simulink model "CLLC_converter_switching_model_closed_loop"  (R2021a)
settings: Solver=VariableStepAuto  StartTime=0.0  StopTime=10.0  MaxStep=1e-9  RelTol=1e-3
undefined symbols (not defined in the file or in its folder): Ion, Lithium
libraries: spsSeriesRLCBranchLib x26, spsMosfetLib x8, spsVoltageMeasurementLib x7, spsCurrentMeasurementLib x6, spsControlledVoltageSourceLib x5, pid_lib x2, spsBatteryLib x1, spsLinearTransformerLib x1, simulink x1, spsVariableResistorLib x1, spspowerguiLib x1
settings Model: Creator=prizm  LastModifiedBy=prizm
settings RTWCC: GenCodeOnly=on

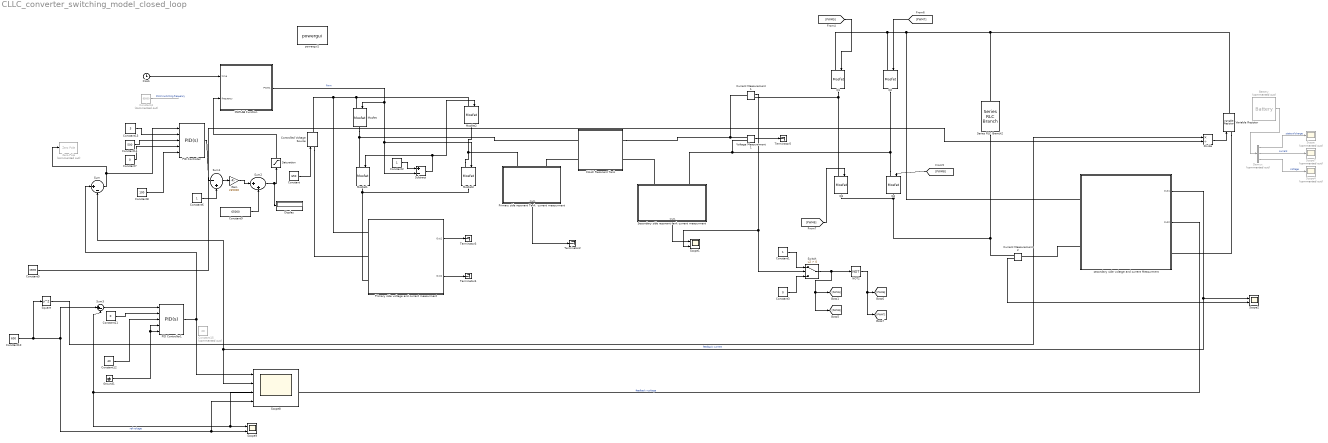
== system CLLC_converter_switching_model_closed_loop ==
  Battery : spsBatteryLib/Battery  Commented=on  BatType=Lithium-Ion  ShowTempParam=off  ThermalPreset=no  ShowAgeParam=off  NomV=662  NomQ=500  SOC=60  Batt_Tr=5e-3  PresetModel=on  MaxQ=500  MinV=496.5  FullV=770.5595  Dis_rate=217.3913  R=0.01324  Normal_OP=452.1739  expZone="[715.2154      24.56522]"  current=[6.5 13 32.5]  Units=Time  Tci=20  NomT=20  T2=-30  MaxQ2=4.8  FullV2=7.1  Normal_OP2=5.655  expZone2="[6.58           1]"  Rca=0.6  ti=2000  Dp=0  Neq0=0  Tsim=1e6  Ta1=25  Qeol=5.4*0.9  Reol=0.013333*1.2  Char_age=[2.3478, 3]  Dis_age=[2.3478, 10]  N1=1500  N2=10500  N3=1000  N4=1400  Ta2=45  N5=950
  "CLLLC Resonant Tank " : Subsystem
  Clock : Clock
  Constant : Constant  Value=650
  Constant1 : Constant
  Constant10 : Constant  Value=600
  Constant11 : Constant  Value=0
  Constant12 : Constant  Value=40
  Constant13 : Constant  Value=3
  Constant14 : Constant  Value=500
  Constant15 : Constant  Commented=on  Value=20  SampleTime=1e-9
  Constant2 : Constant
  Constant3 : Constant  Value=0
  Constant4 : Constant  Commented=on  Value=65000
  Constant5 : Constant  Value=15000  SampleTime=1e-9
  Constant6 : Constant
  Constant7 : Constant  Value=0
  Constant8 : Constant  Value=100
  Constant9 : Constant  Value=65000
  Controlled Voltage Source : spsControlledVoltageSourceLib/Controlled Voltage Source  Initialize=on  Source_Type=DC  Amplitude=0  Phase=0  Frequency=0  Measurements=None
  Current Measurement1 : spsCurrentMeasurementLib/Current Measurement  PhasorSimulation=off  OutputType=Complex  PSBequivalent=0
  Current Measurement2 : spsCurrentMeasurementLib/Current Measurement  PhasorSimulation=off  OutputType=Complex  PSBequivalent=0
  Demux : Demux  Commented=on  Outputs=3
  Display : Display
  Divide : Product  Inputs=*/
  Gain : Gain  Gain=235000
  Ground1 : Ground
  MATLAB Function : MATLAB Function  TreatAsAtomicUnit=on
  Mosfet{,1..3} (4 alike) : spsMosfetLib/Mosfet  Ron=0.1  Lon=0  Rd=0.01  Vfd=2  IC=0  Rs=1e5  Cs=inf  Measurements=off
  NOT2 : Logic  Operator=NOT  IconShape=distinctive  AllPortsSameDT=off  OutDataTypeStr=boolean
  PID Controller : pid_lib/PID Controller  Controller=PID  Form=Parallel  TimeDomain=Continuous-time  UseExternalTs=off  SampleTime=-1  IntegratorMethod=Forward Euler  FilterMethod=Forward Euler  ControllerParametersSource=external  P=0.00014927  I=100  D=0  UseFilter=on  N=100  TunerSelectOption=Frequency Response Based  InitialConditionSource=internal  InitialConditionForIntegrator=0  InitialConditionForFilter=0  DifferentiatorICPrevScaledInput=0  ExternalReset=none  TrackingMode=off  Kt=1  LimitOutput=on  SatLimitsSource=internal  UpperSaturationLimit=1  LowerSaturationLimit=0  LinearizeAsGain=on  AntiWindupMode=clamping  Kb=1  POutMin=[]  POutMax=[]  IOutMin=[]  IOutMax=[]  DOutMin=[]  DOutMax=[]  NOutMin=[]  NOutMax=[]  SumOutMin=[]  SumOutMax=[]  SaturationOutMin=[]  SaturationOutMax=[]  PParamMin=[]  PParamMax=[]  IParamMin=[]  IParamMax=[]  DParamMin=[]  DParamMax=[]  NParamMin=[]  NParamMax=[]  KbParamMin=[]  KbParamMax=[]  KtParamMin=[]  KtParamMax=[]  KbOutMin=[]  KbOutMax=[]  KtOutMin=[]  KtOutMax=[]  IntegratorOutMin=[]  IntegratorOutMax=[]  FilterOutMin=[]  FilterOutMax=[]  SumI1OutMin=[]  SumI1OutMax=[]  SumI2OutMin=[]  SumI2OutMax=[]  SumI3OutMin=[]  SumI3OutMax=[]  SumI4OutMin=[]  SumI4OutMax=[]  SumDOutMin=[]  SumDOutMax=[]  DifferentiatorOutMin=[]  DifferentiatorOutMax=[]  FilterDiffOutCoefMin=[]  FilterDiffOutCoefMax=[]  ReciprocalOutMin=[]  ReciprocalOutMax=[]  SumDenOutMin=[]  SumDenOutMax=[]  SumNumOutMin=[]  SumNumOutMax=[]  DivideOutMin=[]  DivideOutMax=[]  UdiffTsProdOutMin=[]  UdiffTsProdOutMax=[]  NTsProdOutMin=[]  NTsProdOutMax=[]  UintegralTsProdOutMin=[]  UintegralTsProdOutMax=[]  UngainTsProdOutMin=[]  UngainTsProdOutMax=[]  IntegratorContinuousStateAttributes=''  IntegratorStateMustResolveToSignalObject=off  IntegratorRTWStateStorageClass=Auto  FilterContinuousStateAttributes=''  FilterStateMustResolveToSignalObject=off  FilterRTWStateStorageClass=Auto  ParallelPVariant=ExternalParameters  IdealPVariant=Disabled  IVariant=ExternalParameters  DVariant=ExternalParameters  IntegratorVariant=Continuous  SatVariant=Enabled  AWVariant=ContClampingParallel  PCopyVariant=Disabled  TRVariant=Disabled  FdbkBlocksVariant=Forward  IdealPFdbkVariant=Disabled  SatFdbkVariant=Disabled  DerivativeFilterVariant=ContFilter  NVariant=ExternalParameters  NCopyVariant=Disabled  FilterICVariant=InternalICsFilter  IntegratorICVariant=InternalICs  ExternalResetVariant=Disabled  TRSumVariant=Passthrough  SumFdbkVariant=Disabled  SumVariant=Sum_PID  TsampFilterVariant=InternalTs  TsampNgainVariant=Passthrough  TsampIntegralVariant=Passthrough  ExternalSaturationOutDataTypeStr=Inherit: Same as second input
  PID Controller1 : pid_lib/PID Controller  Controller=PID  Form=Parallel  TimeDomain=Continuous-time  UseExternalTs=off  SampleTime=-1  IntegratorMethod=Forward Euler  FilterMethod=Forward Euler  ControllerParametersSource=external  P=0.00014927  I=100  D=0  UseFilter=on  N=100  TunerSelectOption=Frequency Response Based  InitialConditionSource=internal  InitialConditionForIntegrator=0  InitialConditionForFilter=0  DifferentiatorICPrevScaledInput=0  ExternalReset=none  TrackingMode=off  Kt=1  LimitOutput=on  SatLimitsSource=internal  UpperSaturationLimit=30  LowerSaturationLimit=5  LinearizeAsGain=on  AntiWindupMode=clamping  Kb=1  POutMin=[]  POutMax=[]  IOutMin=[]  IOutMax=[]  DOutMin=[]  DOutMax=[]  NOutMin=[]  NOutMax=[]  SumOutMin=[]  SumOutMax=[]  SaturationOutMin=[]  SaturationOutMax=[]  PParamMin=[]  PParamMax=[]  IParamMin=[]  IParamMax=[]  DParamMin=[]  DParamMax=[]  NParamMin=[]  NParamMax=[]  KbParamMin=[]  KbParamMax=[]  KtParamMin=[]  KtParamMax=[]  KbOutMin=[]  KbOutMax=[]  KtOutMin=[]  KtOutMax=[]  IntegratorOutMin=[]  IntegratorOutMax=[]  FilterOutMin=[]  FilterOutMax=[]  SumI1OutMin=[]  SumI1OutMax=[]  SumI2OutMin=[]  SumI2OutMax=[]  SumI3OutMin=[]  SumI3OutMax=[]  SumI4OutMin=[]  SumI4OutMax=[]  SumDOutMin=[]  SumDOutMax=[]  DifferentiatorOutMin=[]  DifferentiatorOutMax=[]  FilterDiffOutCoefMin=[]  FilterDiffOutCoefMax=[]  ReciprocalOutMin=[]  ReciprocalOutMax=[]  SumDenOutMin=[]  SumDenOutMax=[]  SumNumOutMin=[]  SumNumOutMax=[]  DivideOutMin=[]  DivideOutMax=[]  UdiffTsProdOutMin=[]  UdiffTsProdOutMax=[]  NTsProdOutMin=[]  NTsProdOutMax=[]  UintegralTsProdOutMin=[]  UintegralTsProdOutMax=[]  UngainTsProdOutMin=[]  UngainTsProdOutMax=[]  IntegratorContinuousStateAttributes=''  IntegratorStateMustResolveToSignalObject=off  IntegratorRTWStateStorageClass=Auto  FilterContinuousStateAttributes=''  FilterStateMustResolveToSignalObject=off  FilterRTWStateStorageClass=Auto  ParallelPVariant=ExternalParameters  IdealPVariant=Disabled  IVariant=ExternalParameters  DVariant=ExternalParameters  IntegratorVariant=Continuous  SatVariant=Enabled  AWVariant=ContClampingParallel  PCopyVariant=Disabled  TRVariant=Disabled  FdbkBlocksVariant=Forward  IdealPFdbkVariant=Disabled  SatFdbkVariant=Disabled  DerivativeFilterVariant=ContFilter  NVariant=ExternalParameters  NCopyVariant=Disabled  FilterICVariant=InternalICsFilter  IntegratorICVariant=InternalICs  ExternalResetVariant=Disabled  TRSumVariant=Passthrough  SumFdbkVariant=Disabled  SumVariant=Sum_PID  TsampFilterVariant=InternalTs  TsampNgainVariant=Passthrough  TsampIntegralVariant=Passthrough  ExternalSaturationOutDataTypeStr=Inherit: Same as second input
  "Primary side resonant Tank  current measurment " : Subsystem
  "Primary side voltage and current measurment " : Subsystem
  Q{1..4} (4 alike) : spsMosfetLib/Mosfet  Ron=0.1  Lon=0  Rd=0.01  Vfd=2  IC=0  Rs=1e5  Cs=inf  Measurements=off
  Saturation : Saturate  UpperLimit=300000  LowerLimit=60000
  Scope : Scope  Commented=on
  Scope1 : Scope  NumInputPorts=2
  Scope2 : Scope  NumInputPorts=2
  Scope4 : Scope  Commented=on
  Scope7 : Scope  Commented=on
  Scope8 : Scope  NumInputPorts=4
  Scope9 : Scope  NumInputPorts=2
  "Secondary side resonant tank current measurment " : Subsystem
  Series RLC Branch2 : spsSeriesRLCBranchLib/Series RLC Branch  LConnTagsString=__new0  RConnTagsString=__new0  BranchType=C  Resistance=54.0  Inductance=0.2533e-3  SetiL0=off  InitialCurrent=0  Capacitance=10e-6  Setx0=off  InitialVoltage=0  Measurements=None
  Square : Math  Operator=square  SaturateOnIntegerOverflow=on
  Subtract : Sum  Inputs=+-
  Sum : Sum  Inputs=|+-
  Sum1 : Sum  Inputs=|-+
  Sum2 : Sum  Inputs=|++
  Sum3 : Sum  Inputs=|+-
  Switch : Switch  Criteria=u2 > Threshold
  Terminator{2..5} (4 alike) : Terminator
  Variable Resistor : spsVariableResistorLib/Variable Resistor  Rabsmin=1e-3
      settings: SourceProductBaseCode=PS
  Voltage Measurement1 : spsVoltageMeasurementLib/Voltage Measurement  PhasorSimulation=off  OutputType=Complex  PSBequivalent=0
  Zero-Pole : ZeroPole  Commented=on  Zeros=[-3.48e4 -3.48e4]  Poles=[0 -5e4 -3.7699e5]  Gain=[600]
  powergui1 : spspowerguiLib/powergui  Priority=1  SimulationMode=Discrete  SampleTime=1e-9  frequency=60  Iterations=50  frequencyindice=0  Pbase=100e6  ErrMax=1e-4  UnitsV=kV  UnitsW=MW  buscounter=0  FunctionMessages=off  echomessages=off  EnableUseOfTLC=off  CurrentSourceSwitches=off  DisableSnubberDevices=off  DisableRonSwitches=off  DisableVfSwitches=off  DisplayEquations=off  AutomaticDiscreteSolvers=off  SolverType=Tustin/Backward Euler (TBE)  Interpol=off  ExternalGateDelay=off  methode=off  Ts=100  x0status=blocks  SPID=on  SwTol=0  HookPort=off  NonlinearTolerance=1e-4  nMaxIteration=100  ContinueOnMaxIteration=off  RestoreLinks=warning  ResistiveCurrentMeasurement=off  Frange=[0:2:500]  Ylog=off  Xlog=on  ShowGrid=off  save=off  variable=ZData  structure=0  ZoomFFT=off  StartTime=0.0  cycles=1  DisplayStyle=1  fundamental=60  FreqAxis=off  MaxFrequency=1000  frequencyindicesteady=1  RmsSteady=1  display=off
  "secondary side volatge and current Measurment " : Subsystem
  wires:
  Constant/1 -> Controlled Voltage Source/1
  MATLAB Function/1(PWM1) -> Mosfet/1, Mosfet3/1, Subtract/2  "Pwm"
  Constant2/1 -> Subtract/1
  Subtract/1 -> Mosfet2/1, Mosfet1/1
  [PWM7] -> Q2/1
  [PWM6] -> Q3/1
  [PWM8] -> Q4/1
  [PWM5] -> Q1/1
  NOT2/1 -> [PWM6], [PWM7]
  Switch/1 -> [PWM5], [PWM8], NOT2/1
  Current Measurement1/1 -> Scope1/2, Switch/2
  Constant3/1 -> Switch/3
  Constant1/1 -> Switch/1
  Voltage Measurement1/1 -> Terminator5/1
  Sum/1 -> PID Controller/1, Zero-Pole/1
  Constant9/1 -> Sum2/2
  Sum2/1 -> Display/1, Saturation/1
  Ground1/1 -> PID Controller1/5, PID Controller1/4
  Constant10/1 -> Square/1, Sum3/1, Scope8/4, Scope9/2  "ref voltage"
  Sum3/1 -> PID Controller1/1
  Constant11/1 -> PID Controller1/2
  Constant12/1 -> PID Controller1/3
  Sum1/1 -> Gain/1
  Constant6/1 -> Sum1/2
  Saturation/1 -> MATLAB Function/2(frequency)
  Gain/1 -> Sum2/1
  Constant13/1 -> PID Controller/2
  Constant14/1 -> PID Controller/3
  Constant4/1 -> ?  "PWM switching frequency"
  Clock/1 -> MATLAB Function/1(time)
  "Primary side voltage and current measurment "/1(Out1) -> Terminator3/1
  "Primary side voltage and current measurment "/2(Out2) -> Terminator4/1
  "Primary side resonant Tank  current measurment "/1(Out1) -> Terminator2/1
  "Secondary side resonant tank current measurment "/1(Out1) -> Scope1/1
  "secondary side volatge and current Measurment "/2(Out2) -> Sum3/2, Scope8/3, Scope9/1  "feedback vcoltage"
  "secondary side volatge and current Measurment "/1(Out1) -> Scope2/1, Sum/2, Scope8/2  "feedback current"
  Battery/1 -> Demux/1
  Demux/1 -> Scope/1  "state of charge"
  Demux/2 -> Scope7/1  "current"
  Demux/3 -> Scope4/1  "Voltage"
  PID Controller/1 -> Sum1/1
  Constant7/1 -> PID Controller/4
  Constant8/1 -> PID Controller/5
  Divide/1 -> Variable Resistor/1
  PID Controller1/1 -> Sum/1, Scope8/1
  Constant5/1 -> Divide/2
  Square/1 -> Divide/1
  Current Measurement2/1 -> Scope2/2
  connections:
  Controlled Voltage Source/RConn1 -- "Primary side voltage and current measurment "/LConn1 -- Mosfet/LConn1 -- Mosfet2/LConn1
  Mosfet3/RConn1 -- "Primary side voltage and current measurment "/LConn3 -- Mosfet1/RConn1
  Q1/RConn1 -- Q3/LConn1 -- Current Measurement1/RConn1
  Voltage Measurement1/LConn1 -- Current Measurement1/LConn1 -- "CLLLC Resonant Tank "/RConn1
  Controlled Voltage Source/LConn1 -- "Primary side voltage and current measurment "/LConn2
  Mosfet3/LConn1 -- Mosfet2/RConn1 -- "Primary side resonant Tank  current measurment "/LConn1
  Q4/LConn1 -- Q2/RConn1 -- Voltage Measurement1/LConn2 -- "Secondary side resonant tank current measurment "/LConn2
  Q2/LConn1 -- Q1/LConn1 -- Variable Resistor/RConn1 -- Series RLC Branch2/LConn1 -- "secondary side volatge and current Measurment "/LConn1
  Q3/RConn1 -- Current Measurement2/RConn1 -- Series RLC Branch2/RConn1 -- Q4/RConn1
  Variable Resistor/LConn1 -- "secondary side volatge and current Measurment "/RConn1
  Mosfet/RConn1 -- Mosfet1/LConn1 -- "CLLLC Resonant Tank "/LConn1
  "Primary side resonant Tank  current measurment "/LConn2 -- "CLLLC Resonant Tank "/LConn2
  "Secondary side resonant tank current measurment "/LConn1 -- "CLLLC Resonant Tank "/RConn2
  "secondary side volatge and current Measurment "/LConn2 -- Current Measurement2/LConn1

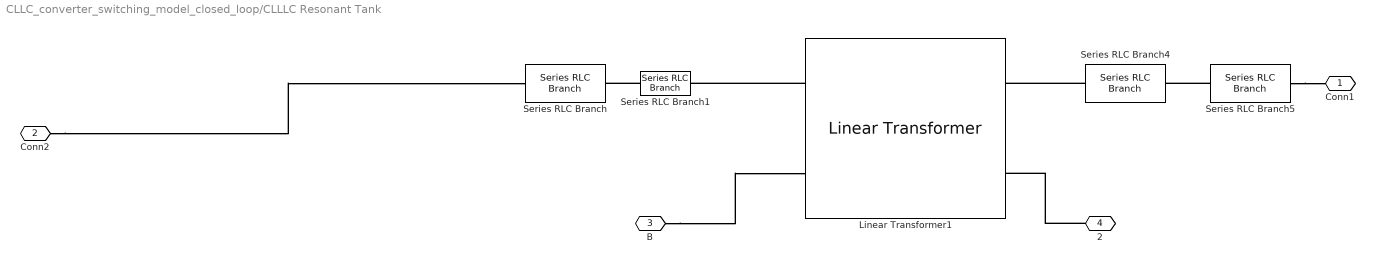
== system CLLC_converter_switching_model_closed_loop/CLLLC Resonant Tank  ==
  Linear Transformer1 : spsLinearTransformerLib/Linear Transformer  UNITS=SI  NominalPower=[15000 60000]  winding1=[500 0.003 10e-9]  winding2=[650 0.003 10e-9]  ThreeWindings=off  winding3=[3.15e+05 0 0]  RmLm=[10e9 100e-6]  Measurements=None  DataType=on
  Series RLC Branch : spsSeriesRLCBranchLib/Series RLC Branch  LConnTagsString=__new0  RConnTagsString=__new0  BranchType=C  Resistance=1  Inductance=1e-3  SetiL0=off  InitialCurrent=0  Capacitance=300e-9  Setx0=off  InitialVoltage=0  Measurements=None
  Series RLC Branch1 : spsSeriesRLCBranchLib/Series RLC Branch  LConnTagsString=__new0  RConnTagsString=__new0  BranchType=L  Resistance=1  Inductance=20e-6  SetiL0=off  InitialCurrent=0  Capacitance=1e-6  Setx0=off  InitialVoltage=0  Measurements=None
  Series RLC Branch4 : spsSeriesRLCBranchLib/Series RLC Branch  LConnTagsString=__new0  RConnTagsString=__new0  BranchType=L  Resistance=1  Inductance=20e-6  SetiL0=off  InitialCurrent=0  Capacitance=1e-6  Setx0=off  InitialVoltage=0  Measurements=None
  Series RLC Branch5 : spsSeriesRLCBranchLib/Series RLC Branch  LConnTagsString=__new0  RConnTagsString=__new0  BranchType=C  Resistance=1  Inductance=1e-3  SetiL0=off  InitialCurrent=0  Capacitance=480e-9  Setx0=off  InitialVoltage=0  Measurements=None
  Conn1 : PMIOPort  Side=Right
  Conn2 : PMIOPort  Port=2  Side=Left
  B : PMIOPort  Port=3  Side=Left
  2 : PMIOPort  Port=4  Side=Right
  connections:
  Linear Transformer1/LConn1 -- Series RLC Branch1/RConn1
  Series RLC Branch5/LConn1 -- Series RLC Branch4/LConn1
  Series RLC Branch1/LConn1 -- Series RLC Branch/RConn1
  Conn2/RConn1 -- Series RLC Branch/LConn1
  B/RConn1 -- Linear Transformer1/LConn2
  2/RConn1 -- Linear Transformer1/RConn2
  Series RLC Branch4/RConn1 -- Linear Transformer1/RConn1
  Series RLC Branch5/RConn1 -- Conn1/RConn1

== system CLLC_converter_switching_model_closed_loop/Primary side resonant Tank  current measurment  ==
  ADC conversion to bits  2 : Subsystem
  CLLLC primary side  side current measurment 2 : Subsystem
  conversion from bits to current1 : Subsystem
  - : PMIOPort  Side=Left
  + : PMIOPort  Port=2  Side=Left
  Out1 : Outport
  wires:
  ADC conversion to bits  2/1(reference) -> conversion from bits to current1/1(reference)
  CLLLC primary side  side current measurment 2/1(v) -> ADC conversion to bits  2/1(v)
  ADC conversion to bits  2/2(Out2) -> conversion from bits to current1/2(In2)
  conversion from bits to current1/1(Out1) -> Out1/1
  connections:
  -/RConn1 -- CLLLC primary side  side current measurment 2/LConn1
  CLLLC primary side  side current measurment 2/LConn2 -- +/RConn1

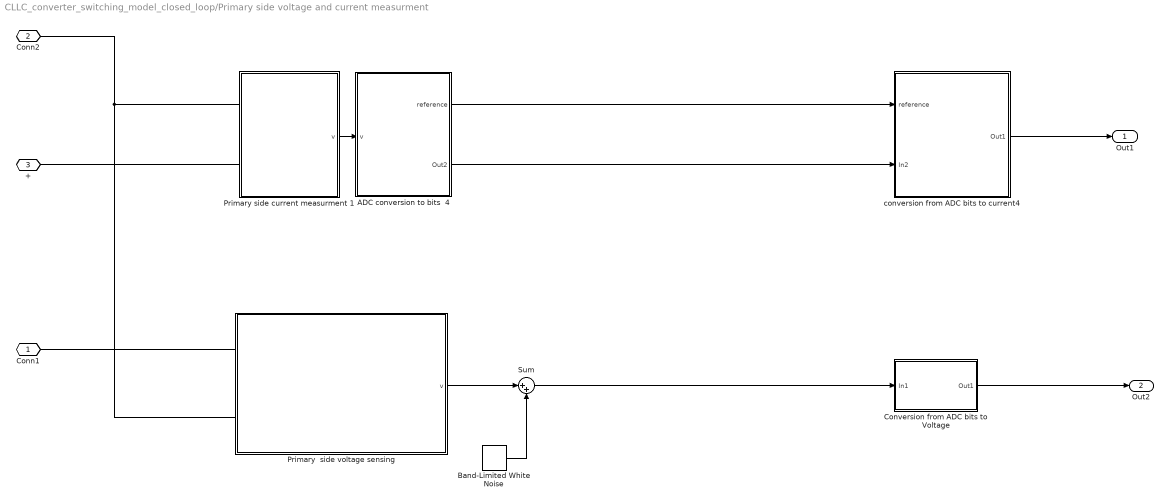
== system CLLC_converter_switching_model_closed_loop/Primary side voltage and current measurment  ==
  ADC conversion to bits  4 : Subsystem
  Band-Limited White Noise : simulink/Sources/Band-Limited White Noise  Cov=[0.1]  Ts=1e-4  seed=[23341]
  "Conversion from ADC bits to Voltage " : Subsystem
  "Primary  side voltage sensing " : Subsystem
  Primary side current measurment 1 : Subsystem
  Sum : Sum  Inputs=|++
  conversion from ADC bits to current4 : Subsystem
  Conn1 : PMIOPort  Side=Left
  Conn2 : PMIOPort  Port=2  Side=Left
  + : PMIOPort  Port=3  Side=Left
  Out1 : Outport
  Out2 : Outport  Port=2
  wires:
  ADC conversion to bits  4/2(Out2) -> conversion from ADC bits to current4/2(In2)
  Primary side current measurment 1/1(v) -> ADC conversion to bits  4/1(v)
  conversion from ADC bits to current4/1(Out1) -> Out1/1
  ADC conversion to bits  4/1(reference) -> conversion from ADC bits to current4/1(reference)
  "Primary  side voltage sensing "/1(v) -> Sum/1
  Band-Limited White Noise/1 -> Sum/2
  Sum/1 -> "Conversion from ADC bits to Voltage "/1(In1)
  "Conversion from ADC bits to Voltage "/1(Out1) -> Out2/1
  connections:
  Conn1/RConn1 -- "Primary  side voltage sensing "/LConn1
  Primary side current measurment 1/LConn2 -- +/RConn1
  Primary side current measurment 1/LConn1 -- Conn2/RConn1 -- "Primary  side voltage sensing "/LConn2

== system CLLC_converter_switching_model_closed_loop/Secondary side resonant tank current measurment  ==
  ADC conversion to bits  1 : Subsystem
  "CLLLC secondary side current measurment " : Subsystem
  conversion from bits to current2 : Subsystem
  - : PMIOPort  Side=Left
  + : PMIOPort  Port=2  Side=Left
  Out1 : Outport
  wires:
  "CLLLC secondary side current measurment "/1(v) -> ADC conversion to bits  1/1(v)
  ADC conversion to bits  1/2(Out2) -> conversion from bits to current2/2(In2)
  ADC conversion to bits  1/1(reference) -> conversion from bits to current2/1(reference)
  conversion from bits to current2/1(Out1) -> Out1/1
  connections:
  "CLLLC secondary side current measurment "/LConn1 -- -/RConn1
  +/RConn1 -- "CLLLC secondary side current measurment "/LConn2

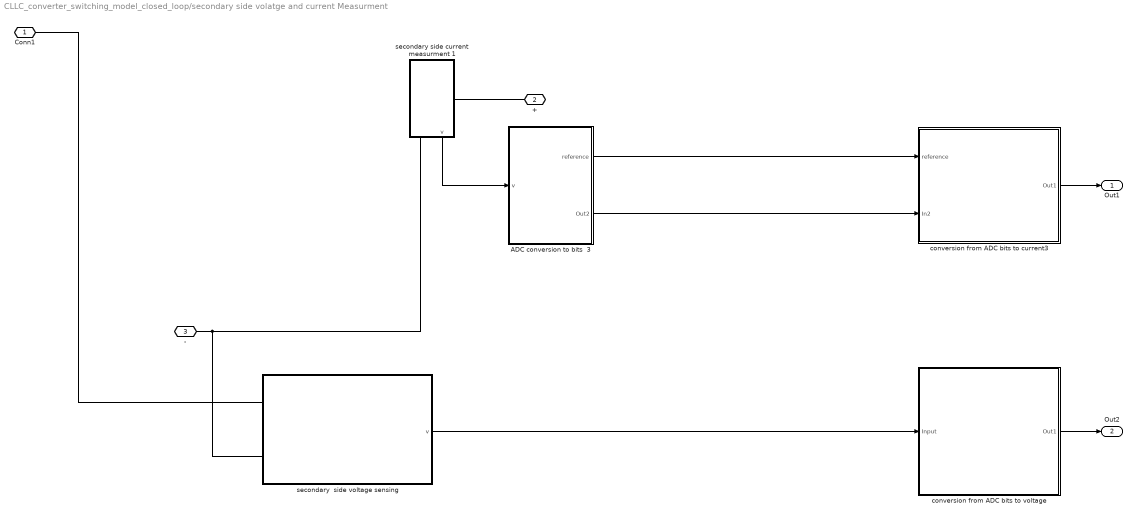
== system CLLC_converter_switching_model_closed_loop/secondary side volatge and current Measurment  ==
  ADC conversion to bits  3 : Subsystem
  conversion from ADC bits to current3 : Subsystem
  "conversion from ADC bits to voltage " : Subsystem
  "secondary  side voltage sensing " : Subsystem
  secondary side current measurment 1 : Subsystem
      settings: PortSchema="{\"entries\":[{\"content\":{\"sides\":[{\"content\":{\"connectorIds\":[]},\"type\":\"ConnectorPlacement.EquallySpacedRectSide\",\"uuid\":\"6682aabd-b4c9-4e26-ac42-b7f4937c9882\"},{\"content\":{\"connectorIds\":[\"RConn1\",\"Out1\"],\"side\":\"RIGHT\"},\"type\":\"ConnectorPlacement.EquallySpacedRectSide\",\"uuid\":\"39693c9e-f70a-4c1a-90ac-326607627fb7\"},{\"content\":{\"connectorIds\":[],\"side\":\"TOP\"},\"type\":\"ConnectorPlacement.EquallySpacedRectSide\",\"uuid\":\"8ffbc9bf-ac02-4293-be03-d78ae118879d\"},{\"content\":{\"connectorIds\":[\"RConn2\"],\"side\":\"BOTTOM\"},\"type\":\"ConnectorPlacement.EquallySpacedRectSide\",\"uuid\":\"c1ea8c00-373b-4bbb-8642-07b7e9a91a0c\"}]},\"type\":\"ConnectorPlacement.EquallySpacedConnector\",\"uuid\":\"fc66d08e-e92c-4509-bb77-625124f73eef\"}],\"packageUris\":[\"http://schema.mathworks.com/mf0/Connector/R2020b\"],\"version\":\"1.0\"}"
  Conn1 : PMIOPort  Side=Left
  + : PMIOPort  Port=2  Side=Right
  - : PMIOPort  Port=3  Side=Left
  Out1 : Outport
  Out2 : Outport  Port=2
  wires:
  secondary side current measurment 1/1(v) -> ADC conversion to bits  3/1(v)
  ADC conversion to bits  3/2(Out2) -> conversion from ADC bits to current3/2(In2)
  ADC conversion to bits  3/1(reference) -> conversion from ADC bits to current3/1(reference)
  conversion from ADC bits to current3/1(Out1) -> Out1/1
  "secondary  side voltage sensing "/1(v) -> "conversion from ADC bits to voltage "/1(Input)
  "conversion from ADC bits to voltage "/1(Out1) -> Out2/1
  connections:
  Conn1/RConn1 -- "secondary  side voltage sensing "/LConn1
  +/RConn1 -- secondary side current measurment 1/RConn2
  -/RConn1 -- "secondary  side voltage sensing "/LConn2 -- secondary side current measurment 1/RConn1

== system CLLC_converter_switching_model_closed_loop/Primary side resonant Tank  current measurment /ADC conversion to bits  2 ==
  v : Inport
  Gain3 : Gain  Gain=(2^12)/3.3
  Gain4 : Gain  Gain=(2^12)/3.3
  rererence voltage : Constant  Value=1.5
  reference : Outport
  Out2 : Outport  Port=2
  wires:
  v/1 -> Gain3/1
  Gain4/1 -> reference/1  "reference"
  rererence voltage/1 -> Gain4/1
  Gain3/1 -> Out2/1

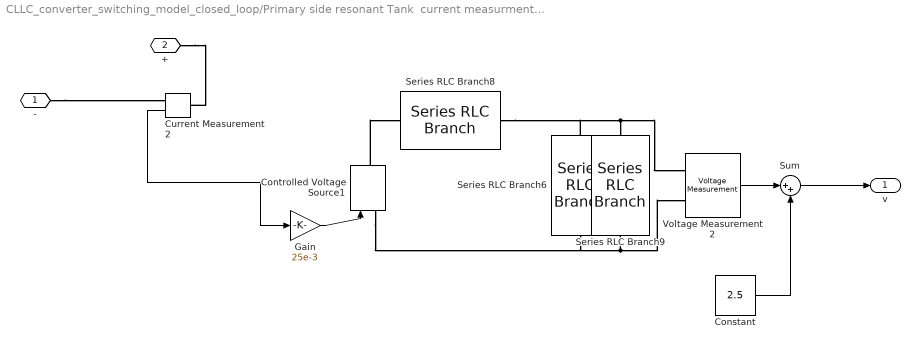
== system CLLC_converter_switching_model_closed_loop/Primary side resonant Tank  current measurment /CLLLC primary side  side current measurment 2 ==
  Constant : Constant  Value=2.5
  Controlled Voltage Source1 : spsControlledVoltageSourceLib/Controlled Voltage Source  Initialize=on  Source_Type=DC  Amplitude=0  Phase=0  Frequency=0  Measurements=None
  Current Measurement2 : spsCurrentMeasurementLib/Current Measurement  PhasorSimulation=off  OutputType=Complex  PSBequivalent=0
  Gain : Gain  Gain=25e-3
  Series RLC Branch6 : spsSeriesRLCBranchLib/Series RLC Branch  LConnTagsString=__new0  RConnTagsString=__new0  BranchType=R  Resistance=15e3  Inductance=0.2533e-3  SetiL0=off  InitialCurrent=0  Capacitance=1e-6  Setx0=off  InitialVoltage=0  Measurements=None
  Series RLC Branch8 : spsSeriesRLCBranchLib/Series RLC Branch  LConnTagsString=__new0  RConnTagsString=__new0  BranchType=R  Resistance=10e3  Inductance=0.2533e-3  SetiL0=off  InitialCurrent=0  Capacitance=1e-6  Setx0=off  InitialVoltage=0  Measurements=None
  Series RLC Branch9 : spsSeriesRLCBranchLib/Series RLC Branch  LConnTagsString=__new0  RConnTagsString=__new0  BranchType=C  Resistance=54.0  Inductance=0.2533e-3  SetiL0=off  InitialCurrent=0  Capacitance=220e-12  Setx0=off  InitialVoltage=0  Measurements=None
  Sum : Sum  Inputs=|++
  Voltage Measurement2 : spsVoltageMeasurementLib/Voltage Measurement  PhasorSimulation=off  OutputType=Complex  PSBequivalent=0
  - : PMIOPort  Side=Left
  + : PMIOPort  Port=2  Side=Left
  v : Outport
  wires:
  Gain/1 -> Controlled Voltage Source1/1
  Current Measurement2/1 -> Gain/1
  Voltage Measurement2/1 -> Sum/1
  Constant/1 -> Sum/2
  Sum/1 -> v/1
  connections:
  Series RLC Branch9/RConn1 -- Series RLC Branch6/LConn1 -- Controlled Voltage Source1/LConn1 -- Voltage Measurement2/LConn2
  Controlled Voltage Source1/RConn1 -- Series RLC Branch8/RConn1
  Series RLC Branch9/LConn1 -- Series RLC Branch6/RConn1 -- Series RLC Branch8/LConn1 -- Voltage Measurement2/LConn1
  +/RConn1 -- Current Measurement2/LConn1
  -/RConn1 -- Current Measurement2/RConn1

== system CLLC_converter_switching_model_closed_loop/Primary side resonant Tank  current measurment /conversion from bits to current1 ==
  reference : Inport
  In2 : Inport  Port=2
  Gain : Gain  Gain=40
  Gain3 : Gain  Gain=25/15
  Gain4 : Gain  Gain=3.3/(2^12)
  Minus : Sum  Inputs=-+
  Out1 : Outport
  wires:
  In2/1 -> Minus/2
  Minus/1 -> Gain4/1
  reference/1 -> Minus/1
  Gain4/1 -> Gain3/1
  Gain3/1 -> Gain/1
  Gain/1 -> Out1/1

== system CLLC_converter_switching_model_closed_loop/Primary side voltage and current measurment /ADC conversion to bits  4 ==
  v : Inport
  Gain3 : Gain  Gain=(2^12)/3.3
  Gain4 : Gain  Gain=(2^12)/3.3
  rererence voltage : Constant  Value=1.5
  reference : Outport
  Out2 : Outport  Port=2
  wires:
  v/1 -> Gain3/1
  Gain4/1 -> reference/1  "reference"
  rererence voltage/1 -> Gain4/1
  Gain3/1 -> Out2/1

== system CLLC_converter_switching_model_closed_loop/Primary side voltage and current measurment /Conversion from ADC bits to Voltage  ==
  In1 : Inport
  "1KHz LPF Butter worth IIR " : Subsystem  Tag=FilterWizardSubSystem
      settings: ErrorFcn=dspFilterRealizedInBasicElemsAlgLoopErrFcnCallback
  Gain1 : Gain  Gain=477.1
  Gain3 : Gain  Gain=3.3/(2^12)
  Out1 : Outport
  wires:
  Gain1/1 -> Out1/1
  Gain3/1 -> Gain1/1
  In1/1 -> "1KHz LPF Butter worth IIR "/1(Input)
  "1KHz LPF Butter worth IIR "/1(Output) -> Gain3/1

== system CLLC_converter_switching_model_closed_loop/Primary side voltage and current measurment /Primary  side voltage sensing  ==
  Gain : Gain  Gain=(2^12)/3.3
  Series RLC Branch6 : spsSeriesRLCBranchLib/Series RLC Branch  LConnTagsString=__new0  RConnTagsString=__new0  BranchType=R  Resistance=10e6  Inductance=0.2533e-3  SetiL0=off  InitialCurrent=0  Capacitance=1e-6  Setx0=off  InitialVoltage=0  Measurements=None
  Series RLC Branch7 : spsSeriesRLCBranchLib/Series RLC Branch  LConnTagsString=__new0  RConnTagsString=__new0  BranchType=R  Resistance=21e3  Inductance=0.2533e-3  SetiL0=off  InitialCurrent=0  Capacitance=1e-6  Setx0=off  InitialVoltage=0  Measurements=None
  Series RLC Branch8 : spsSeriesRLCBranchLib/Series RLC Branch  LConnTagsString=__new0  RConnTagsString=__new0  BranchType=R  Resistance=10e3  Inductance=0.2533e-3  SetiL0=off  InitialCurrent=0  Capacitance=1e-6  Setx0=off  InitialVoltage=0  Measurements=None
  Series RLC Branch9 : spsSeriesRLCBranchLib/Series RLC Branch  LConnTagsString=__new0  RConnTagsString=__new0  BranchType=C  Resistance=54.0  Inductance=0.2533e-3  SetiL0=off  InitialCurrent=0  Capacitance=100e-12  Setx0=off  InitialVoltage=0  Measurements=None
  Voltage Measurement2 : spsVoltageMeasurementLib/Voltage Measurement  PhasorSimulation=off  OutputType=Complex  PSBequivalent=0
  Conn1 : PMIOPort  Side=Left
  Conn2 : PMIOPort  Port=2  Side=Left
  v : Outport
  wires:
  Voltage Measurement2/1 -> Gain/1
  Gain/1 -> v/1
  connections:
  Voltage Measurement2/LConn2 -- Series RLC Branch9/RConn1 -- Series RLC Branch7/RConn1 -- Conn2/RConn1
  Voltage Measurement2/LConn1 -- Series RLC Branch8/LConn1 -- Series RLC Branch9/LConn1
  Series RLC Branch6/RConn1 -- Series RLC Branch7/LConn1 -- Series RLC Branch8/RConn1
  Conn1/RConn1 -- Series RLC Branch6/LConn1

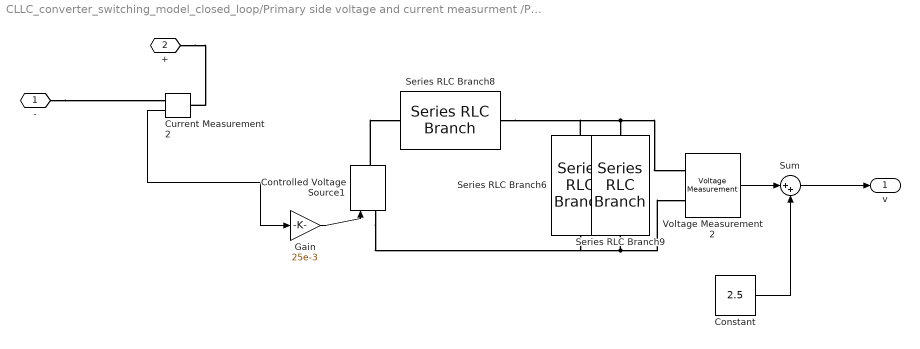
== system CLLC_converter_switching_model_closed_loop/Primary side voltage and current measurment /Primary side current measurment 1 ==
  Constant : Constant  Value=2.5
  Controlled Voltage Source1 : spsControlledVoltageSourceLib/Controlled Voltage Source  Initialize=on  Source_Type=DC  Amplitude=0  Phase=0  Frequency=0  Measurements=None
  Current Measurement2 : spsCurrentMeasurementLib/Current Measurement  PhasorSimulation=off  OutputType=Complex  PSBequivalent=0
  Gain : Gain  Gain=25e-3
  Series RLC Branch6 : spsSeriesRLCBranchLib/Series RLC Branch  LConnTagsString=__new0  RConnTagsString=__new0  BranchType=R  Resistance=15e3  Inductance=0.2533e-3  SetiL0=off  InitialCurrent=0  Capacitance=1e-6  Setx0=off  InitialVoltage=0  Measurements=None
  Series RLC Branch8 : spsSeriesRLCBranchLib/Series RLC Branch  LConnTagsString=__new0  RConnTagsString=__new0  BranchType=R  Resistance=10e3  Inductance=0.2533e-3  SetiL0=off  InitialCurrent=0  Capacitance=1e-6  Setx0=off  InitialVoltage=0  Measurements=None
  Series RLC Branch9 : spsSeriesRLCBranchLib/Series RLC Branch  LConnTagsString=__new0  RConnTagsString=__new0  BranchType=C  Resistance=54.0  Inductance=0.2533e-3  SetiL0=off  InitialCurrent=0  Capacitance=220e-12  Setx0=off  InitialVoltage=0  Measurements=None
  Sum : Sum  Inputs=|++
  Voltage Measurement2 : spsVoltageMeasurementLib/Voltage Measurement  PhasorSimulation=off  OutputType=Complex  PSBequivalent=0
  - : PMIOPort  Side=Left
  + : PMIOPort  Port=2  Side=Left
  v : Outport
  wires:
  Gain/1 -> Controlled Voltage Source1/1
  Current Measurement2/1 -> Gain/1
  Voltage Measurement2/1 -> Sum/1
  Constant/1 -> Sum/2
  Sum/1 -> v/1
  connections:
  Series RLC Branch9/RConn1 -- Series RLC Branch6/LConn1 -- Controlled Voltage Source1/LConn1 -- Voltage Measurement2/LConn2
  Controlled Voltage Source1/RConn1 -- Series RLC Branch8/RConn1
  Series RLC Branch9/LConn1 -- Series RLC Branch6/RConn1 -- Series RLC Branch8/LConn1 -- Voltage Measurement2/LConn1
  +/RConn1 -- Current Measurement2/LConn1
  -/RConn1 -- Current Measurement2/RConn1

== system CLLC_converter_switching_model_closed_loop/Primary side voltage and current measurment /conversion from ADC bits to current4 ==
  reference : Inport
  In2 : Inport  Port=2
  Gain : Gain  Gain=40
  Gain3 : Gain  Gain=25/15
  Gain4 : Gain  Gain=3.3/(2^12)
  Minus : Sum  Inputs=-+
  Out1 : Outport
  wires:
  In2/1 -> Minus/2
  Minus/1 -> Gain4/1
  reference/1 -> Minus/1
  Gain4/1 -> Gain3/1
  Gain3/1 -> Gain/1
  Gain/1 -> Out1/1

== system CLLC_converter_switching_model_closed_loop/Secondary side resonant tank current measurment /ADC conversion to bits  1 ==
  v : Inport
  Gain3 : Gain  Gain=(2^12)/3.3
  Gain4 : Gain  Gain=(2^12)/3.3
  rererence voltage : Constant  Value=1.5
  reference : Outport
  Out2 : Outport  Port=2
  wires:
  v/1 -> Gain3/1
  Gain4/1 -> reference/1  "reference"
  rererence voltage/1 -> Gain4/1
  Gain3/1 -> Out2/1

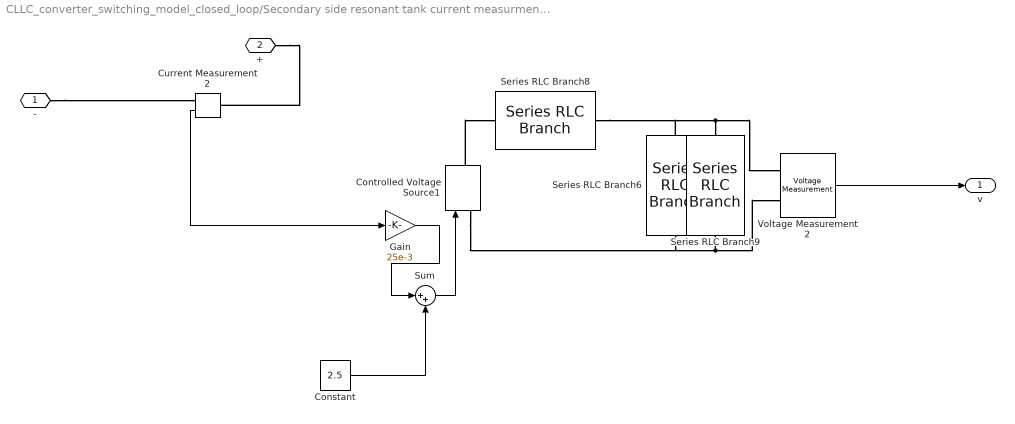
== system CLLC_converter_switching_model_closed_loop/Secondary side resonant tank current measurment /CLLLC secondary side current measurment  ==
  Constant : Constant  Value=2.5
  Controlled Voltage Source1 : spsControlledVoltageSourceLib/Controlled Voltage Source  Initialize=on  Source_Type=DC  Amplitude=0  Phase=0  Frequency=0  Measurements=None
  Current Measurement2 : spsCurrentMeasurementLib/Current Measurement  PhasorSimulation=off  OutputType=Complex  PSBequivalent=0
  Gain : Gain  Gain=25e-3
  Series RLC Branch6 : spsSeriesRLCBranchLib/Series RLC Branch  LConnTagsString=__new0  RConnTagsString=__new0  BranchType=R  Resistance=15e3  Inductance=0.2533e-3  SetiL0=off  InitialCurrent=0  Capacitance=1e-6  Setx0=off  InitialVoltage=0  Measurements=None
  Series RLC Branch8 : spsSeriesRLCBranchLib/Series RLC Branch  LConnTagsString=__new0  RConnTagsString=__new0  BranchType=R  Resistance=10e3  Inductance=0.2533e-3  SetiL0=off  InitialCurrent=0  Capacitance=1e-6  Setx0=off  InitialVoltage=0  Measurements=None
  Series RLC Branch9 : spsSeriesRLCBranchLib/Series RLC Branch  LConnTagsString=__new0  RConnTagsString=__new0  BranchType=C  Resistance=54.0  Inductance=0.2533e-3  SetiL0=off  InitialCurrent=0  Capacitance=220e-12  Setx0=off  InitialVoltage=0  Measurements=None
  Sum : Sum  Inputs=|++
  Voltage Measurement2 : spsVoltageMeasurementLib/Voltage Measurement  PhasorSimulation=off  OutputType=Complex  PSBequivalent=0
  - : PMIOPort  Side=Left
  + : PMIOPort  Port=2  Side=Left
  v : Outport
  wires:
  Gain/1 -> Sum/1
  Current Measurement2/1 -> Gain/1
  Voltage Measurement2/1 -> v/1
  Constant/1 -> Sum/2
  Sum/1 -> Controlled Voltage Source1/1
  connections:
  Series RLC Branch9/RConn1 -- Series RLC Branch6/LConn1 -- Controlled Voltage Source1/LConn1 -- Voltage Measurement2/LConn2
  Controlled Voltage Source1/RConn1 -- Series RLC Branch8/RConn1
  Series RLC Branch9/LConn1 -- Series RLC Branch6/RConn1 -- Series RLC Branch8/LConn1 -- Voltage Measurement2/LConn1
  +/RConn1 -- Current Measurement2/LConn1
  -/RConn1 -- Current Measurement2/RConn1

== system CLLC_converter_switching_model_closed_loop/Secondary side resonant tank current measurment /conversion from bits to current2 ==
  reference : Inport
  In2 : Inport  Port=2
  Gain : Gain  Gain=40
  Gain3 : Gain  Gain=25/15
  Gain4 : Gain  Gain=3.3/(2^12)
  Minus : Sum  Inputs=-+
  Out1 : Outport
  wires:
  In2/1 -> Minus/2
  Minus/1 -> Gain4/1
  Gain4/1 -> Gain3/1
  Gain3/1 -> Gain/1
  Gain/1 -> Out1/1
  reference/1 -> Minus/1

== system CLLC_converter_switching_model_closed_loop/secondary side volatge and current Measurment /ADC conversion to bits  3 ==
  v : Inport
  Gain3 : Gain  Gain=(2^12)/3.3
  Gain4 : Gain  Gain=(2^12)/3.3
  rererence voltage : Constant  Value=1.5
  reference : Outport
  Out2 : Outport  Port=2
  wires:
  v/1 -> Gain3/1
  Gain4/1 -> reference/1  "reference"
  rererence voltage/1 -> Gain4/1
  Gain3/1 -> Out2/1

== system CLLC_converter_switching_model_closed_loop/secondary side volatge and current Measurment /conversion from ADC bits to current3 ==
  reference : Inport
  In2 : Inport  Port=2
  "20 KHz Lpf butterworth " : Subsystem  Tag=FilterWizardSubSystem  Commented=on
      settings: ErrorFcn=dspFilterRealizedInBasicElemsAlgLoopErrFcnCallback
  Gain : Gain  Gain=40
  Gain3 : Gain  Gain=25/15
  Gain4 : Gain  Gain=3.3/(2^12)
  Minus : Sum  Inputs=-+
  Out1 : Outport
  wires:
  In2/1 -> Minus/2
  reference/1 -> Minus/1
  Gain4/1 -> Gain3/1
  Gain3/1 -> Gain/1
  Gain/1 -> Out1/1
  Minus/1 -> Gain4/1

== system CLLC_converter_switching_model_closed_loop/secondary side volatge and current Measurment /conversion from ADC bits to voltage  ==
  Input : Inport
  "1KHz LPF Butter worth IIR " : Subsystem  Tag=FilterWizardSubSystem  Commented=on
      settings: ErrorFcn=dspFilterRealizedInBasicElemsAlgLoopErrFcnCallback
  Gain2 : Gain  Gain=477.1
  Gain3 : Gain  Gain=3.3/(2^12)
  Out1 : Outport
  wires:
  Gain3/1 -> Gain2/1
  Gain2/1 -> Out1/1
  Input/1 -> Gain3/1

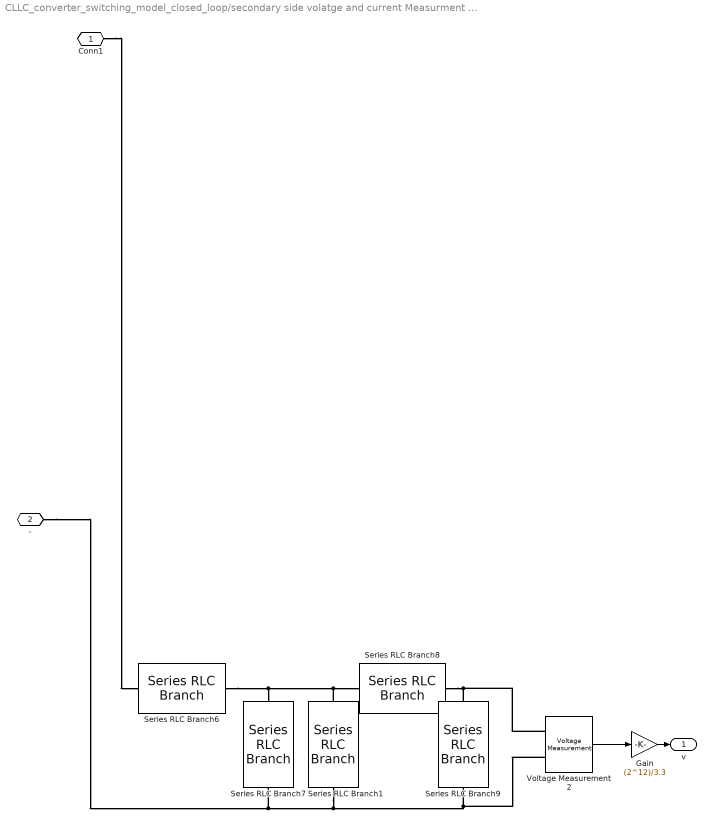
== system CLLC_converter_switching_model_closed_loop/secondary side volatge and current Measurment /secondary  side voltage sensing  ==
  Gain : Gain  Gain=(2^12)/3.3
  Series RLC Branch1 : spsSeriesRLCBranchLib/Series RLC Branch  LConnTagsString=__new0  RConnTagsString=__new0  BranchType=C  Resistance=54.0  Inductance=0.2533e-3  SetiL0=off  InitialCurrent=0  Capacitance=0.2e-12  Setx0=off  InitialVoltage=0  Measurements=None
  Series RLC Branch6 : spsSeriesRLCBranchLib/Series RLC Branch  LConnTagsString=__new0  RConnTagsString=__new0  BranchType=R  Resistance=10e6  Inductance=0.2533e-3  SetiL0=off  InitialCurrent=0  Capacitance=1e-6  Setx0=off  InitialVoltage=0  Measurements=None
  Series RLC Branch7 : spsSeriesRLCBranchLib/Series RLC Branch  LConnTagsString=__new0  RConnTagsString=__new0  BranchType=R  Resistance=21e3  Inductance=0.2533e-3  SetiL0=off  InitialCurrent=0  Capacitance=1e-6  Setx0=off  InitialVoltage=0  Measurements=None
  Series RLC Branch8 : spsSeriesRLCBranchLib/Series RLC Branch  LConnTagsString=__new0  RConnTagsString=__new0  BranchType=R  Resistance=10e3  Inductance=0.2533e-3  SetiL0=off  InitialCurrent=0  Capacitance=1e-6  Setx0=off  InitialVoltage=0  Measurements=None
  Series RLC Branch9 : spsSeriesRLCBranchLib/Series RLC Branch  LConnTagsString=__new0  RConnTagsString=__new0  BranchType=C  Resistance=54.0  Inductance=0.2533e-3  SetiL0=off  InitialCurrent=0  Capacitance=100e-12  Setx0=off  InitialVoltage=0  Measurements=None
  Voltage Measurement2 : spsVoltageMeasurementLib/Voltage Measurement  PhasorSimulation=off  OutputType=Complex  PSBequivalent=0
  Conn1 : PMIOPort  Side=Left
  - : PMIOPort  Port=2  Side=Left
  v : Outport
  wires:
  Voltage Measurement2/1 -> Gain/1
  Gain/1 -> v/1
  connections:
  Series RLC Branch7/RConn1 -- Series RLC Branch1/RConn1 -- Voltage Measurement2/LConn2 -- Series RLC Branch9/RConn1 -- -/RConn1
  Series RLC Branch8/LConn1 -- Voltage Measurement2/LConn1 -- Series RLC Branch9/LConn1
  Series RLC Branch6/RConn1 -- Series RLC Branch1/LConn1 -- Series RLC Branch8/RConn1 -- Series RLC Branch7/LConn1
  Conn1/RConn1 -- Series RLC Branch6/LConn1

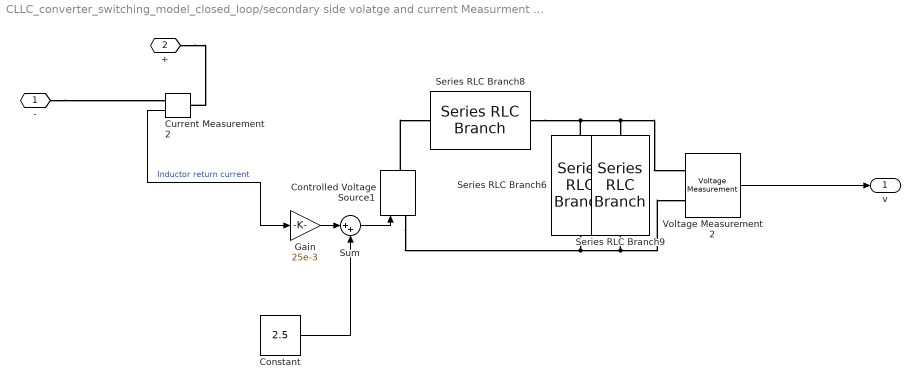
== system CLLC_converter_switching_model_closed_loop/secondary side volatge and current Measurment /secondary side current measurment 1 ==
  Constant : Constant  Value=2.5
  Controlled Voltage Source1 : spsControlledVoltageSourceLib/Controlled Voltage Source  Initialize=on  Source_Type=DC  Amplitude=0  Phase=0  Frequency=0  Measurements=None
  Current Measurement2 : spsCurrentMeasurementLib/Current Measurement  PhasorSimulation=off  OutputType=Complex  PSBequivalent=0
  Gain : Gain  Gain=25e-3
  Series RLC Branch6 : spsSeriesRLCBranchLib/Series RLC Branch  LConnTagsString=__new0  RConnTagsString=__new0  BranchType=R  Resistance=15e3  Inductance=0.2533e-3  SetiL0=off  InitialCurrent=0  Capacitance=1e-6  Setx0=off  InitialVoltage=0  Measurements=None
  Series RLC Branch8 : spsSeriesRLCBranchLib/Series RLC Branch  LConnTagsString=__new0  RConnTagsString=__new0  BranchType=R  Resistance=10e3  Inductance=0.2533e-3  SetiL0=off  InitialCurrent=0  Capacitance=1e-6  Setx0=off  InitialVoltage=0  Measurements=None
  Series RLC Branch9 : spsSeriesRLCBranchLib/Series RLC Branch  LConnTagsString=__new0  RConnTagsString=__new0  BranchType=C  Resistance=54.0  Inductance=0.2533e-3  SetiL0=off  InitialCurrent=0  Capacitance=220e-12  Setx0=off  InitialVoltage=0  Measurements=None
  Sum : Sum  Inputs=|++
  Voltage Measurement2 : spsVoltageMeasurementLib/Voltage Measurement  PhasorSimulation=off  OutputType=Complex  PSBequivalent=0
  - : PMIOPort  Side=Right
  + : PMIOPort  Port=2  Side=Right
  v : Outport
  wires:
  Current Measurement2/1 -> Gain/1  "Inductor return current"
  Voltage Measurement2/1 -> v/1
  Constant/1 -> Sum/2
  Gain/1 -> Sum/1
  Sum/1 -> Controlled Voltage Source1/1
  connections:
  Controlled Voltage Source1/LConn1 -- Series RLC Branch6/LConn1 -- Voltage Measurement2/LConn2 -- Series RLC Branch9/RConn1
  Controlled Voltage Source1/RConn1 -- Series RLC Branch8/RConn1
  Series RLC Branch8/LConn1 -- Series RLC Branch6/RConn1 -- Voltage Measurement2/LConn1 -- Series RLC Branch9/LConn1
  +/RConn1 -- Current Measurement2/LConn1
  -/RConn1 -- Current Measurement2/RConn1

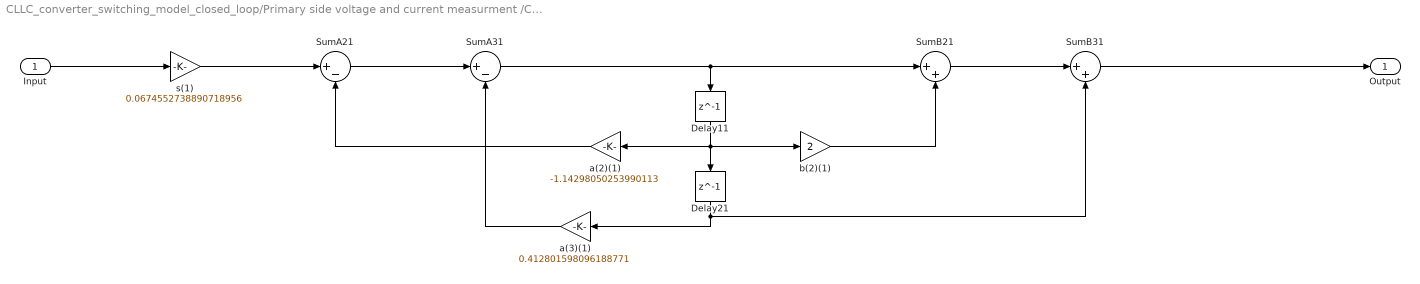
== system CLLC_converter_switching_model_closed_loop/Primary side voltage and current measurment /Conversion from ADC bits to Voltage /1KHz LPF Butter worth IIR  ==
  Input : Inport
  Delay11 : Delay  DelayLength=1  InitialCondition=0
  Delay21 : Delay  DelayLength=1  InitialCondition=0
  SumA21 : Sum  Inputs=|+-  RndMeth=Nearest  SaturateOnIntegerOverflow=on  OutDataTypeStr=Inherit: Same as first input
  SumA31 : Sum  Inputs=|+-  RndMeth=Nearest  SaturateOnIntegerOverflow=on  OutDataTypeStr=Inherit: Same as first input
  SumB21 : Sum  Inputs=|++  RndMeth=Nearest  SaturateOnIntegerOverflow=on  OutDataTypeStr=Inherit: Same as first input
  SumB31 : Sum  Inputs=|++  RndMeth=Nearest  SaturateOnIntegerOverflow=on  OutDataTypeStr=Inherit: Same as first input
  a(2)(1) : Gain  Gain=-1.14298050253990113  ParamDataTypeStr=double  RndMeth=Nearest  SaturateOnIntegerOverflow=on  OutDataTypeStr=Inherit: Same as input
  a(3)(1) : Gain  Gain=0.412801598096188771  ParamDataTypeStr=double  RndMeth=Nearest  SaturateOnIntegerOverflow=on  OutDataTypeStr=Inherit: Same as input
  b(2)(1) : Gain  Gain=2  ParamDataTypeStr=double  RndMeth=Nearest  SaturateOnIntegerOverflow=on  OutDataTypeStr=Inherit: Same as input
  s(1) : Gain  Gain=0.0674552738890718956  ParamDataTypeStr=double  RndMeth=Nearest  SaturateOnIntegerOverflow=on  OutDataTypeStr=Inherit: Same as input
  Output : Outport
  wires:
  Input/1 -> s(1)/1
  s(1)/1 -> SumA21/1
  SumA21/1 -> SumA31/1
  SumA31/1 -> SumB21/1, Delay11/1
  SumB21/1 -> SumB31/1
  SumB31/1 -> Output/1
  a(2)(1)/1 -> SumA21/2
  Delay11/1 -> a(2)(1)/1, b(2)(1)/1, Delay21/1
  b(2)(1)/1 -> SumB21/2
  a(3)(1)/1 -> SumA31/2
  Delay21/1 -> a(3)(1)/1, SumB31/2

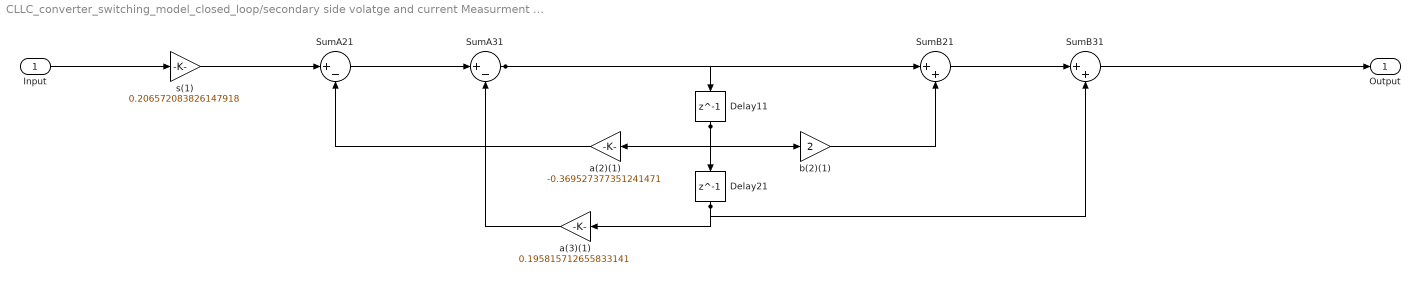
== system CLLC_converter_switching_model_closed_loop/secondary side volatge and current Measurment /conversion from ADC bits to current3/20 KHz Lpf butterworth  ==
  Input : Inport
  Delay11 : Delay  DelayLength=1  InitialCondition=0
  Delay21 : Delay  DelayLength=1  InitialCondition=0
  SumA21 : Sum  Inputs=|+-  RndMeth=Nearest  SaturateOnIntegerOverflow=on  OutDataTypeStr=Inherit: Same as first input
  SumA31 : Sum  Inputs=|+-  RndMeth=Nearest  SaturateOnIntegerOverflow=on  OutDataTypeStr=Inherit: Same as first input
  SumB21 : Sum  Inputs=|++  RndMeth=Nearest  SaturateOnIntegerOverflow=on  OutDataTypeStr=Inherit: Same as first input
  SumB31 : Sum  Inputs=|++  RndMeth=Nearest  SaturateOnIntegerOverflow=on  OutDataTypeStr=Inherit: Same as first input
  a(2)(1) : Gain  Gain=-0.369527377351241471  ParamDataTypeStr=double  RndMeth=Nearest  SaturateOnIntegerOverflow=on  OutDataTypeStr=Inherit: Same as input
  a(3)(1) : Gain  Gain=0.195815712655833141  ParamDataTypeStr=double  RndMeth=Nearest  SaturateOnIntegerOverflow=on  OutDataTypeStr=Inherit: Same as input
  b(2)(1) : Gain  Gain=2  ParamDataTypeStr=double  RndMeth=Nearest  SaturateOnIntegerOverflow=on  OutDataTypeStr=Inherit: Same as input
  s(1) : Gain  Gain=0.206572083826147918  ParamDataTypeStr=double  RndMeth=Nearest  SaturateOnIntegerOverflow=on  OutDataTypeStr=Inherit: Same as input
  Output : Outport
  wires:
  Input/1 -> s(1)/1
  s(1)/1 -> SumA21/1
  SumA21/1 -> SumA31/1
  SumA31/1 -> SumB21/1, Delay11/1
  SumB21/1 -> SumB31/1
  SumB31/1 -> Output/1
  a(2)(1)/1 -> SumA21/2
  Delay11/1 -> a(2)(1)/1, b(2)(1)/1, Delay21/1
  b(2)(1)/1 -> SumB21/2
  a(3)(1)/1 -> SumA31/2
  Delay21/1 -> a(3)(1)/1, SumB31/2

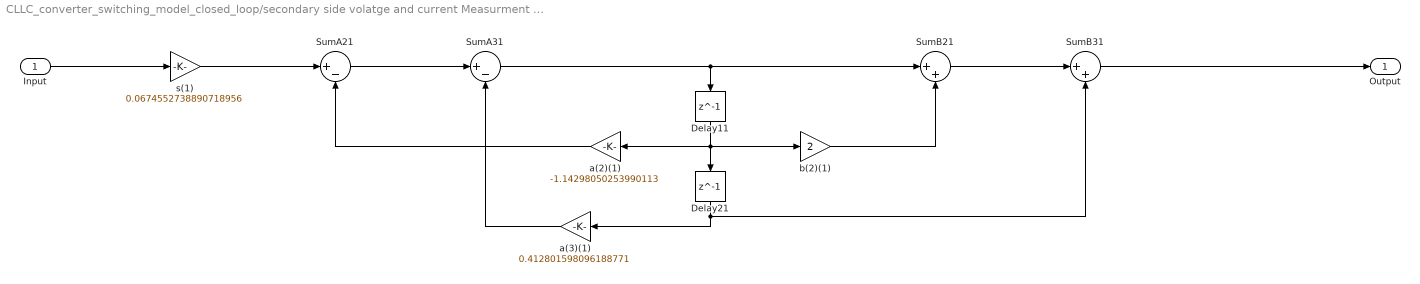
== system CLLC_converter_switching_model_closed_loop/secondary side volatge and current Measurment /conversion from ADC bits to voltage /1KHz LPF Butter worth IIR  ==
  Input : Inport
  Delay11 : Delay  DelayLength=1  InitialCondition=0
  Delay21 : Delay  DelayLength=1  InitialCondition=0
  SumA21 : Sum  Inputs=|+-  RndMeth=Nearest  SaturateOnIntegerOverflow=on  OutDataTypeStr=Inherit: Same as first input
  SumA31 : Sum  Inputs=|+-  RndMeth=Nearest  SaturateOnIntegerOverflow=on  OutDataTypeStr=Inherit: Same as first input
  SumB21 : Sum  Inputs=|++  RndMeth=Nearest  SaturateOnIntegerOverflow=on  OutDataTypeStr=Inherit: Same as first input
  SumB31 : Sum  Inputs=|++  RndMeth=Nearest  SaturateOnIntegerOverflow=on  OutDataTypeStr=Inherit: Same as first input
  a(2)(1) : Gain  Gain=-1.14298050253990113  ParamDataTypeStr=double  RndMeth=Nearest  SaturateOnIntegerOverflow=on  OutDataTypeStr=Inherit: Same as input
  a(3)(1) : Gain  Gain=0.412801598096188771  ParamDataTypeStr=double  RndMeth=Nearest  SaturateOnIntegerOverflow=on  OutDataTypeStr=Inherit: Same as input
  b(2)(1) : Gain  Gain=2  ParamDataTypeStr=double  RndMeth=Nearest  SaturateOnIntegerOverflow=on  OutDataTypeStr=Inherit: Same as input
  s(1) : Gain  Gain=0.0674552738890718956  ParamDataTypeStr=double  RndMeth=Nearest  SaturateOnIntegerOverflow=on  OutDataTypeStr=Inherit: Same as input
  Output : Outport
  wires:
  Input/1 -> s(1)/1
  s(1)/1 -> SumA21/1
  SumA21/1 -> SumA31/1
  SumA31/1 -> SumB21/1, Delay11/1
  SumB21/1 -> SumB31/1
  SumB31/1 -> Output/1
  a(2)(1)/1 -> SumA21/2
  Delay11/1 -> a(2)(1)/1, b(2)(1)/1, Delay21/1
  b(2)(1)/1 -> SumB21/2
  a(3)(1)/1 -> SumA31/2
  Delay21/1 -> a(3)(1)/1, SumB31/2

== matlab function CLLC_converter_switching_model_closed_loop/MATLAB Function ==
  data: time input; frequency input; PWM1 output
function PWM1  = fcn(time,frequency)
Tswitching = 1/frequency; 
PWM1 = 0;
y1= mod(time,Tswitching);
if y1<Tswitching/2
    PWM1 = 1; 
end
